simulink model "pilote_hydraulique_Stateflow_1_dashboard"  (R2018a)
settings: Solver=ode23t  StartTime=0.0  StopTime=1500  RelTol=1e-3  EnableMultiTasking=on
undefined symbols (not defined in the file): sigbuilder_block, X, Y, Z
libraries: sm_lib x295, fl_lib x24, nesl_utility x13, sh_lib x5, simulink x1
(part 7 of 7)

== stateflow chart pilote_hydraulique_Stateflow_1_dashboard/Simulink et StateFlow/Chart ==
  settings: sampleTime=0.1
  state Commande_de_cap
    state Gestion_voyant [parallel]
      during:
      voyant_rouge=in(Suivi_de_cap.Correction_de_cap);
      settings: executionOrder=1
    state Suivi_de_cap [parallel]
      settings: executionOrder=2
      state Correction_de_cap
        during:
        cons_barre=(cons_cap-mes_cap);
      state Temporisation
        entry:
        cons_barre=0;
      state Pause
        entry:
        cons_barre=0;
      (default) -> Pause
      Temporisation -> Correction_de_cap [order 2] : after(20,sec)
      Pause -> Temporisation : [abs(cons_cap-mes_cap)>0.1]
      Temporisation -> Pause [order 1] : [abs(cons_cap-mes_cap)<0.1]
      Correction_de_cap -> Pause : [abs(cons_cap-mes_cap)<0.05]
  (default) -> Commande_de_cap
  data: cons_cap input; mes_cap input; cons_barre output double; voyant_rouge output double
